simulink model "vehicle_simulationV2"  (R2020a)
settings: Solver=ode1  StartTime=0.0  StopTime=500  FixedStep=0.1  RelTol=1e-3
undefined symbols (not defined in the file): HDBK, MIL, serial
libraries: powerlib_meascontrol x7, aerolibconvert2 x5, aerolibatmos2 x3, instrumentlib x3, dspsrcs4 x2, simulink x1
(part 6 of 6)

== matlab function vehicle_simulationV2/Simulation/RLV/Force X ==
  data: y output; CrossSec input; rho input; V input; droque input; main input; trig input; abort input; In input; M input
function y = fcn(CrossSec,rho,V, droque, main, trig, abort, In, M)

Cd_cross = 1.25;
if droque ~= 0 && main ~= 0 && abort == 0
    y = In/M;
elseif trig == 1 && (droque ~= 1 ||  main ~= 1) 
    y = 0.5*rho*V*abs(V)*Cd_cross*CrossSec/M;
else
    y = 0;
end

== matlab function vehicle_simulationV2/Simulation/RLV/Force Z ==
  data: y output; CrossSec input; rho input; V input; droque input; main input; trig input; abort input; In input; M input
function y = fcn(CrossSec,rho,V, droque, main, trig, abort, In, M)

Cd_cross = 1.25;
if droque ~= 0 && main ~= 0 && abort == 0
    y = In/M;
elseif trig == 1 && (droque ~= 1 ||  main ~= 1) 
    y = 0.5*rho*V*abs(V)*Cd_cross*CrossSec/M;
else
    y = 0;
end

== matlab function vehicle_simulationV2/Simulation/RLV/Force Pitch ==
  data: theta input; y output; Cd input; CrossSec input; rho input; V input; droque input; main input; trig input; abort input
function y = fcn(theta, Cd, CrossSec,rho,V, droque, main, trig, abort)

if trig == 1 && droque ~= 0 && main ~= 0 && abort == 0
    y = 0.5*rho*CrossSec*V*abs(V)*Cd*sin(theta);
else
    y = 0;
end

== matlab function vehicle_simulationV2/Simulation/RLV/Force Yaw ==
  data: theta input; y output; Cd input; CrossSec input; rho input; V input; droque input; main input; trig input; abort input
function y = fcn(theta, Cd, CrossSec,rho,V, droque, main, trig, abort)

if trig == 1 && droque ~= 0 && main ~= 0 && abort == 0
    y = 0.5*rho*CrossSec*V*abs(V)*Cd*sin(theta);
else
    y = 0;
end

== matlab function vehicle_simulationV2/Simulation/Flight Triggers ==
  data: ignition_trig input; y output; abort_trig input
function y = fcn(ignition_trig,abort_trig)

if ignition_trig == 1 || abort_trig == 1
    y = 0;
else
    y = 1;
end

== matlab function vehicle_simulationV2/Simulation/Balloon Dynamics/balloon acceleration X ==
  data: Cd input; y output; V input; VwindX input; m input; air_rho input; Vol input
function y = fcn(Cd,V,VwindX,m,air_rho,Vol)

Ac = pi*(3/(4*pi)*Vol)^2/3;
F_wind = 0.5*Cd*VwindX*abs(VwindX)*air_rho*Ac;
F_drag = 0.5*air_rho*V*abs(V)*Ac*Cd;
y= F_wind/m - F_drag/m;

== matlab function vehicle_simulationV2/Simulation/Balloon Dynamics/balloon acceleration Y ==
  data: Cd input; y output; V input; VwindX input; m input; air_rho input; Vol input
function y = fcn(Cd,V,VwindX,m,air_rho,Vol)

Ac = pi*(3/(4*pi)*Vol)^2/3;
F_wind = 0.5*Cd*VwindX*abs(VwindX)*air_rho*Ac;
F_drag = 0.5*air_rho*V*abs(V)*Ac*Cd;
y= F_wind/m - F_drag/m;

== matlab function vehicle_simulationV2/Simulation/Mass of Balloon ==
  data: thickness input; y output; Area input; density input
function y = fcn(thickness,Area,density)

y = thickness*Area*density;

== matlab function vehicle_simulationV2/Simulation/RLV/Force Axial ==
  data: Thrust input; y output; Cd input; CrossSec input; rho input; V input; droque input; main input; trig input; abort input
function y = fcn(Thrust, Cd, CrossSec,rho,V, droque, main, trig, abort)
 
if trig == 1 && droque ~= 0 && main ~= 0 && abort == 0
    y = Thrust - 0.5*rho*CrossSec*V^2*Cd;
else
    y = 0;
end
